simulink model "PV_inc"  (R2020b)
settings: Solver=FixedStepAuto  StartTime=0.0  StopTime=0.3  FixedStep=1e-6  RelTol=1e-3
libraries: powerlib x17, re_lib x4, powerlib_meascontrol x1, simulink x1
settings Model: SimulationMode=accelerator  Creator=11383  LastModifiedBy=Administrator
settings DataIOCC: ReturnWorkspaceOutputs=off
settings DebuggingCC: ArithmeticOperatorsInVariantConditions=warning
settings SFSimCC: SimUseLocalCustomCode=off  CustomCodeUndefinedFunction=UseInterfaceOnly
settings RTWCC: RTWUseLocalCustomCode=off
settings CodeAppCC: StateflowObjectComments=on
settings SimscapeCC: SimscapeNormalizeSystem=off

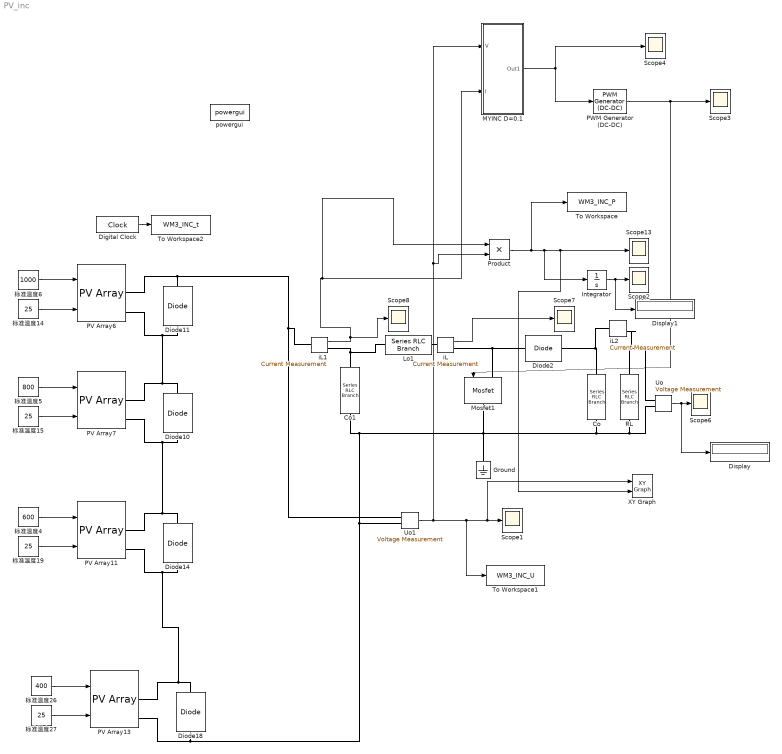
== system PV_inc ==
  Co : powerlib/Elements/Series RLC Branch  LConnTagsString=__new0  RConnTagsString=__new0  BranchType=C  Resistance=1e-4  Inductance=50e-3  SetiL0=off  InitialCurrent=0  Capacitance=9e-5  Setx0=off  InitialVoltage=0  Measurements=None
  Co1 : powerlib/Elements/Series RLC Branch  LConnTagsString=__new0  RConnTagsString=__new0  BranchType=C  Resistance=1e-4  Inductance=50e-3  SetiL0=off  InitialCurrent=0  Capacitance=200e-5  Setx0=off  InitialVoltage=0  Measurements=None
  Digital Clock : DigitalClock  SampleTime=-1
  Diode{10..11,14,18} (4 alike) : powerlib/Power Electronics/Diode  Ron=0.001  Lon=0  Vf=0.8  IC=0  UseSnubber=off  Rs=inf  Cs=250e-9  Measurements=off
  Diode2 : powerlib/Power Electronics/Diode  Ron=0.001  Lon=0  Vf=0.001  IC=0  UseSnubber=off  Rs=inf  Cs=inf  Measurements=off
  Display : Display
  Display1 : Display
  Ground : powerlib/Elements/Ground  LConnTagsString=a
  Integrator : Integrator
  Lo1 : powerlib/Elements/Series RLC Branch  LConnTagsString=__new0  RConnTagsString=__new0  BranchType=L  Resistance=0.1  Inductance=2e-3  SetiL0=off  InitialCurrent=0  Capacitance=1e-12  Setx0=off  InitialVoltage=0  Measurements=None
  MYINC D=0.1 : Subsystem
  Mosfet1 : powerlib/Power Electronics/Mosfet  Ron=0.001  Lon=0  Rd=0.0001  Vfd=0  IC=0  Rs=1e8  Cs=inf  Measurements=off
  PV Array{6..7,11,13} (4 alike) : re_lib/Solar/PV Array  Npar=1  Nser=1  PlotType=array @ 1000 W/m2 & specified temperatures  S_vec="[ 1000  500  100 ]"  Temp_C_vec="[ 45 25  ]"  ModuleName=User-defined  PlotWhenSelected=off  Pm=120.75  Ncell=16  Voc=22  Isc=7.5  Vm=17.5  Im=6.9  beta_Voc_pc=-0.36099  alpha_Isc_pc=0.102  beta_Voc=-0.079418  alpha_Isc=0.00765  IL=7.6829  I0=2.1898e-10  nI=2.2089  Rsh=50.0358  Rs=0.26399  RobustModel=off  RobustCellTemperature=313.3991  BAL=off  Tc=1e-6  Tfilter=5e-5
  PWM Generator (DC-DC) : powerlib_meascontrol/Pulse & Signal Generators/PWM Generator (DC-DC)  Fsw=5000  Ts=5e-6
  Product : Product
  RL : powerlib/Elements/Series RLC Branch  LConnTagsString=__new0  RConnTagsString=__new0  BranchType=R  Resistance=33  Inductance=50e-3  SetiL0=off  InitialCurrent=0  Capacitance=1e-12  Setx0=off  InitialVoltage=0  Measurements=None
  Scope{1..4,6..8,13} (8 alike) : Scope
  To Workspace : ToWorkspace  VariableName=WM3_INC_P  SampleTime=-1
  To Workspace1 : ToWorkspace  VariableName=WM3_INC_U  SampleTime=-1
  To Workspace2 : ToWorkspace  VariableName=WM3_INC_t  SampleTime=-1
  Uo : powerlib/Measurements/Voltage Measurement  PhasorSimulation=off  OutputType=Complex  PSBequivalent=0
  Uo1 : powerlib/Measurements/Voltage Measurement  PhasorSimulation=off  OutputType=Complex  PSBequivalent=0
  XY Graph : simulink/Sinks/XY Graph  xmin=0  xmax=88  ymin=0  ymax=500  st=-1
  iL : powerlib/Measurements/Current Measurement  PhasorSimulation=off  OutputType=Complex  PSBequivalent=0
  iL1 : powerlib/Measurements/Current Measurement  PhasorSimulation=off  OutputType=Complex  PSBequivalent=0
  iL2 : powerlib/Measurements/Current Measurement  PhasorSimulation=off  OutputType=Complex  PSBequivalent=0
  powergui : powerlib/powergui  SimulationMode=Discrete  SampleTime=1e-6  frequency=60  Iterations=50  frequencyindice=0  Pbase=100e6  ErrMax=1e-4  UnitsV=kV  UnitsW=MW  buscounter=0  FunctionMessages=off  echomessages=off  EnableUseOfTLC=off  CurrentSourceSwitches=off  DisableSnubberDevices=off  DisableRonSwitches=off  DisableVfSwitches=off  DisplayEquations=off  AutomaticDiscreteSolvers=off  SolverType=Tustin  Interpol=off  ExternalGateDelay=off  methode=off  Ts=0  x0status=blocks  SPID=off  SwTol=0  HookPort=off  NonlinearTolerance=0  nMaxIteration=15  ContinueOnMaxIteration=off  RestoreLinks=warning  ResistiveCurrentMeasurement=off  Frange=[0:2:500]  Ylog=off  Xlog=on  ShowGrid=off  save=off  variable=ZData  structure=0  ZoomFFT=on  StartTime=0.0  cycles=1  DisplayStyle=1  fundamental=60  FreqAxis=off  MaxFrequency=1000  frequencyindicesteady=1  RmsSteady=1  display=off
  标准温度{14..15,19,27} (4 alike) : Constant  Value=25  SampleTime=0.001
  标准温度26 : Constant  Value=400  SampleTime=0.001
  标准温度4 : Constant  Value=600  SampleTime=0.001
  标准温度5 : Constant  Value=800  SampleTime=0.001
  标准温度6 : Constant  Value=1000  SampleTime=0.001
  wires:
  Uo/1 -> Display/1, Scope6/1
  PWM Generator (DC-DC)/1 -> Mosfet1/1, Scope3/1
  MYINC D=0.1/1(Out1) -> PWM Generator (DC-DC)/1, Scope4/1
  Product/1 -> To Workspace/1, Integrator/1, XY Graph/2, Scope13/1
  Uo1/1 -> To Workspace1/1, XY Graph/1, Scope1/1, MYINC D=0.1/1("V "), Product/2
  标准温度14/1 -> PV Array6/2
  标准温度15/1 -> PV Array7/2
  标准温度19/1 -> PV Array11/2
  标准温度26/1 -> PV Array13/1
  标准温度27/1 -> PV Array13/2
  标准温度6/1 -> PV Array6/1
  标准温度5/1 -> PV Array7/1
  标准温度4/1 -> PV Array11/1
  iL/1 -> Scope7/1
  iL1/1 -> Scope8/1, MYINC D=0.1/2(I), Product/1
  Digital Clock/1 -> To Workspace2/1
  Integrator/1 -> Display1/1, Scope2/1
  connections:
  Uo/LConn1 -- iL2/RConn1 -- RL/RConn1
  Mosfet1/LConn1 -- Diode2/LConn1 -- iL/RConn1
  iL1/RConn1 -- Co1/LConn1 -- Lo1/LConn1
  PV Array6/RConn1 -- Uo1/LConn1 -- iL1/LConn1 -- Diode11/RConn1
  Diode11/LConn1 -- Diode10/RConn1 -- PV Array7/RConn1 -- PV Array6/RConn2
  PV Array11/RConn1 -- Diode10/LConn1 -- PV Array7/RConn2 -- Diode14/RConn1
  Diode14/LConn1 -- Diode18/RConn1 -- PV Array13/RConn1 -- PV Array11/RConn2
  Diode18/LConn1 -- PV Array13/RConn2 -- Uo1/LConn2 -- Mosfet1/RConn1 -- Ground/LConn1 -- Co/RConn1 -- RL/LConn1 -- Uo/LConn2 -- Co1/RConn1
  iL/LConn1 -- Lo1/RConn1
  Co/LConn1 -- iL2/LConn1 -- Diode2/RConn1

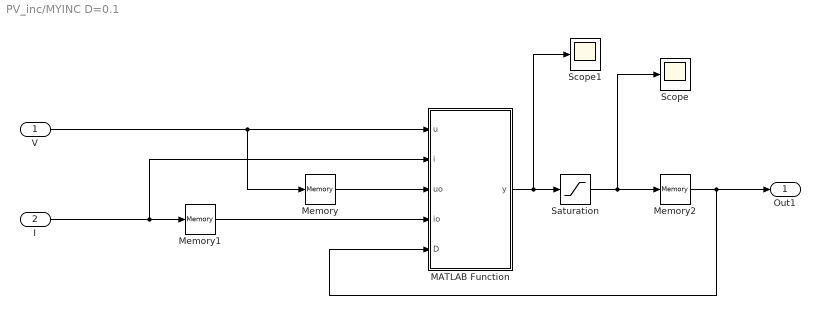
== system PV_inc/MYINC D=0.1 ==
  "V " : Inport
  I : Inport  Port=2
  MATLAB Function : MATLAB Function  TreatAsAtomicUnit=on
  Memory : Memory
  Memory1 : Memory
  Memory2 : Memory
  Saturation : Saturate  UpperLimit=0.9  LowerLimit=0.1
  Scope : Scope
  Scope1 : Scope
  Out1 : Outport  VectorParamsAs1DForOutWhenUnconnected=off
  wires:
  Saturation/1 -> Memory2/1, Scope/1
  MATLAB Function/1(y) -> Saturation/1, Scope1/1
  Memory2/1 -> Out1/1, MATLAB Function/5(D)
  Memory1/1 -> MATLAB Function/4(io)
  I/1 -> MATLAB Function/2(i), Memory1/1
  Memory/1 -> MATLAB Function/3(uo)
  "V "/1 -> MATLAB Function/1(u), Memory/1

== matlab function PV_inc/MYINC D=0.1/MATLAB Function ==
  data: u input; y output; i input; uo input; io input; D input
function y = MYMPP(u,i,uo,io,D)
persistent m; %稳态前两步采样时间控制量
if isempty(m)
    m=0.01;
end
du=u-uo;
di=i-io;
dp=(u*i)-(uo*io);
d=0.001;
if du==0
    if di==0
    m=D;
    else
        if di>0
            m=D-d;
        else m=D+d;
        end
    end
else
    if di/du== -(i/u)
    m=D;
    else
        if di/du> -(i/u)
        m=D-d;
        else m=D+d;
        end
    end
end
y = m;
end
